simulink model "modell"  (R2014b)
settings: Solver=ode45  StartTime=0.0  StopTime=10.0  RelTol=1e-3
values from neighbouring files (symbols this model uses):
  A = [-0.0017 0.0413 -5.3257 -9.7565 ... (first row only)    [AC12.m]    (also in HE5.m = [0 0 0 0.9986 0.0534 0 0 0)
  B = [0.2086 -0.0005 -0.0271 ... (first row only)    [AC12.m]    (also in HE5.m = [0 0 0 0)
  C = [0 0 57.2958 0 ... (first row only)    [AC12.m]    (also in HE5.m = [ 0 0 1 0 0 0 0 0)
undefined symbols (not defined in the file or in its folder): D
libraries: simulink x1
settings Model: Creator=KK  LastModifiedBy=KK

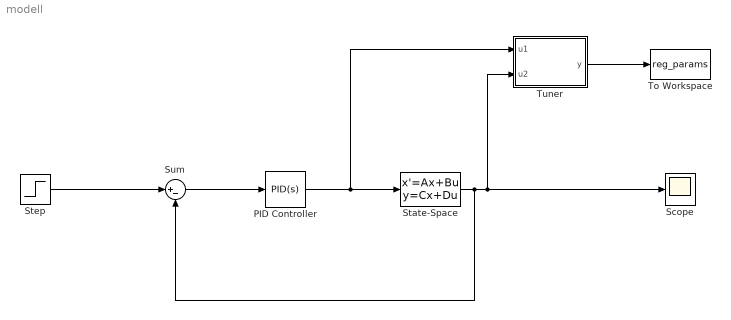
== system modell ==
  PID Controller : simulink/Continuous/PID Controller  Controller=PID  TimeDomain=Continuous-time  SampleTime=-1  IntegratorMethod=Forward Euler  FilterMethod=Forward Euler  Form=Parallel  P=1  I=1  D=0  N=100  InitialConditionSource=internal  InitialConditionForIntegrator=0  InitialConditionForFilter=0  ExternalReset=none  LimitOutput=off  UpperSaturationLimit=inf  LowerSaturationLimit=-inf  LinearizeAsGain=on  AntiWindupMode=none  Kb=1  TrackingMode=off  Kt=1  PParamMin=[]  PParamMax=[]  IParamMin=[]  IParamMax=[]  DParamMin=[]  DParamMax=[]  NParamMin=[]  NParamMax=[]  KbParamMin=[]  KbParamMax=[]  KtParamMin=[]  KtParamMax=[]  POutMin=[]  POutMax=[]  IOutMin=[]  IOutMax=[]  DOutMin=[]  DOutMax=[]  NOutMin=[]  NOutMax=[]  KbOutMin=[]  KbOutMax=[]  KtOutMin=[]  KtOutMax=[]  IntegratorOutMin=[]  IntegratorOutMax=[]  FilterOutMin=[]  FilterOutMax=[]  SumOutMin=[]  SumOutMax=[]  SumI1OutMin=[]  SumI1OutMax=[]  SumI2OutMin=[]  SumI2OutMax=[]  SumI3OutMin=[]  SumI3OutMax=[]  SumDOutMin=[]  SumDOutMax=[]  SaturationOutMin=[]  SaturationOutMax=[]  IntegratorContinuousStateAttributes=''  IntegratorStateMustResolveToSignalObject=off  IntegratorRTWStateStorageClass=Auto  FilterContinuousStateAttributes=''  FilterStateMustResolveToSignalObject=off  FilterRTWStateStorageClass=Auto  DifferentiatorICPrevScaledInput=0  DifferentiatorOutMin=[]  DifferentiatorOutMax=[]  UseFilter=on
  Scope : Scope
  State-Space : StateSpace  A=A  B=B  C=C  D=D  X0=0
  Step : Step  SampleTime=0
  Sum : Sum  Inputs=|+-
  To Workspace : ToWorkspace  VariableName=reg_params  SaveFormat=Timeseries  SampleTime=-1
  Tuner : MATLAB Function  TreatAsAtomicUnit=on
  wires:
  Step/1 -> Sum/1
  Sum/1 -> PID Controller/1
  PID Controller/1 -> Tuner/1(u1), State-Space/1
  State-Space/1 -> Tuner/2(u2), Scope/1, Sum/2
  Tuner/1(y) -> To Workspace/1

== matlab function modell/Tuner ==
  data: u1 input; y output; u2 input
function y = fcn(u1, u2)
%#codegen

y = u;
